simulink model "Computer"  (R2018b)
settings: Solver=ode4  StartTime=0.0  StopTime=SimEndTime  FixedStep=TimeStep  RelTol=1e-3
model workspace (MATLAB code in the model file):
  | CON = Simulink.Parameter;
  | CON.DataType = 'Bus: Bus_CON';
  | CON.Value = Simulink.Bus.createMATLABStruct('Bus_CON');
undefined symbols (not defined in the file): computer_dt
settings Model: ParameterArgumentNames=CON  OrderedModelArguments=off  Creator=Ethan  LastModifiedBy=Ethan
settings ModelReferenceCC: ModelReferenceNumInstancesAllowed=Single

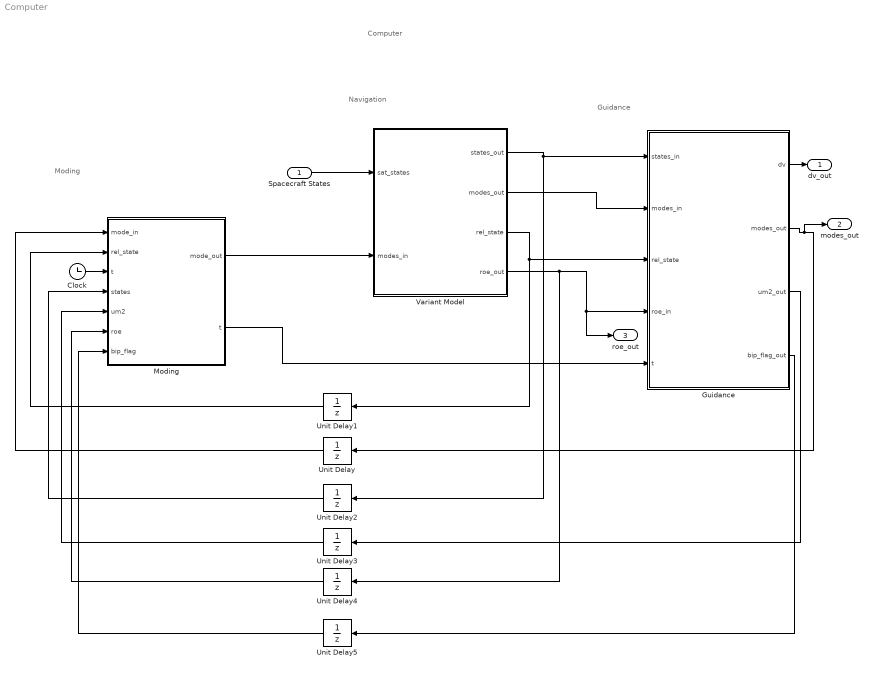
== system Computer ==
  note: Navigation
  note: Computer
  note: Moding
  note: Guidance
  Spacecraft States : Inport  OutDataTypeStr=Bus: Bus_outputs
  Clock : Clock
  Guidance : MATLAB Function  TreatAsAtomicUnit=on  SystemSampleTime=computer_dt
  Moding : MATLAB Function  TreatAsAtomicUnit=on  SystemSampleTime=computer_dt
  Unit Delay{,1..5} (6 alike) : UnitDelay  SampleTime=-1
  Variant Model : Subsystem  Variant=on
  dv_out : Outport  PortDimensions=3
  modes_out : Outport  Port=2  OutDataTypeStr=Bus: Bus_modes
  roe_out : Outport  Port=3  OutDataTypeStr=Bus: Bus_roe
  wires:
  Spacecraft States/1 -> Variant Model/1(sat_states)
  Variant Model/1(states_out) -> Unit Delay2/1, Guidance/1(states_in)
  Guidance/1(dv) -> dv_out/1
  Clock/1 -> Moding/3("t ")
  Moding/1(mode_out) -> Variant Model/2(modes_in)
  Variant Model/2(modes_out) -> Guidance/2(modes_in)
  Guidance/2(modes_out) -> modes_out/1, Unit Delay/1
  Unit Delay/1 -> Moding/1(mode_in)
  Variant Model/3(rel_state) -> Guidance/3(rel_state), Unit Delay1/1
  Unit Delay1/1 -> Moding/2(rel_state)
  Variant Model/4(roe_out) -> Unit Delay4/1, roe_out/1, Guidance/4(roe_in)
  Unit Delay2/1 -> Moding/4(states)
  Guidance/3(um2_out) -> Unit Delay3/1
  Unit Delay3/1 -> Moding/5(um2)
  Unit Delay4/1 -> Moding/6(roe)
  Moding/2(t) -> Guidance/5(t)
  Guidance/4(bip_flag_out) -> Unit Delay5/1
  Unit Delay5/1 -> Moding/7(bip_flag)

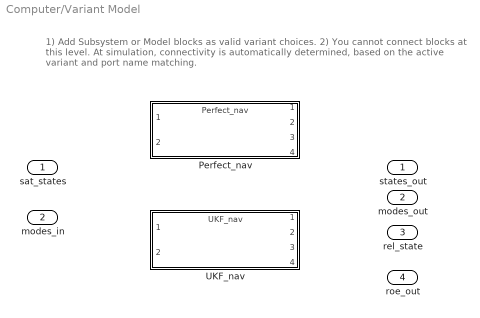
== system Computer/Variant Model ==
  note: 1) Add Subsystem or Model blocks as valid variant choices.
      | 2) You cannot connect blocks at this level. At simulation, connectivity is automatically
      | determined, based on the active variant and port name matching.
  sat_states : Inport  OutDataTypeStr=Bus: Bus_outputs
  modes_in : Inport  Port=2  OutDataTypeStr=Bus: Bus_modes
  Perfect_nav : ModelReference  DisableCoverage=on  ModelNameDialog=Perfect_nav  ParameterArgumentNames=CON  ParameterArgumentValues=CON  UsingDefaultArgumentValue=0  SimulationMode=Normal  VariantControl=Nav_variant  ModelReferenceVersion=1.97
  UKF_nav : ModelReference  ModelNameDialog=UKF_nav  ParameterArgumentNames=CON  ParameterArgumentValues=CON  UsingDefaultArgumentValue=0  SimulationMode=Normal  VariantControl=UKF_variant  ModelReferenceVersion=1.166
  states_out : Outport  OutDataTypeStr=Bus: Bus_outputs
  modes_out : Outport  Port=2  OutDataTypeStr=Bus: Bus_modes
  rel_state : Outport  Port=3
  roe_out : Outport  Port=4  OutDataTypeStr=Bus: Bus_roe

== matlab function Computer/Guidance ==
  data: states_in input; modes_in input Bus: Bus_modes; rel_state input; roe_in input; t input; dv output; CON parameter; modes_out output Bus: Bus_modes; um2_out output; bip_flag_out output
function [dv, modes_out, um2_out, bip_flag_out] = guid_bound_motion(states_in, modes_in, rel_state, roe_in, t, CON)
modes_out = modes_in;
dv = zeros(3, 1);
chief = states_in.NXS_out;
deputy = states_in.astro_out;
i2lvlh = rv2RTN(deputy.r_i, deputy.v_i);

persistent dv_old dv2 um2 xi bip_flag hold_start da de
if isempty(dv_old)
    dv_old = zeros(3, 1);
    dv2 = zeros(3, 1);
    um2 = 999;
    xi = 1000;
    bip_flag = 0;
    hold_start = 0;
    da = -10000;
    de = zeros(2,1);
end

%% New ROE Guidance
if modes_in.guid == 1 % go to 0.5 km relative
    
    [a_c] = ECI2OE(chief.r_i, chief.v_i, CON.mu);
    [~, ~, ~, ~, ~, ~, ud] = ECI2OE(deputy.r_i, deputy.v_i, CON.mu);
    %     if da == -10000
    da = -roe_in.da + 0.491/a_c;
    de = [-roe_in.dey;-roe_in.dex];
    %     end
    %     de = [0; 0];
    if xi == 1000
        xi = atan2(de(2), de(1));
        if xi < 0
            xi = xi + 2 * pi;
        end
    end
    
    um2 = xi + pi;
    if um2 > 2 * pi
        um2 = um2 - 2 * pi;
    elseif um2 < 0
        um2 = um2 + 2 * pi;
    end
    if dv_old ~= zeros(3, 1)
        modes_out.guid = 2;
        dv = zeros(3, 1);
    else
        if abs(ud * pi/180 - xi) < 1e-4
            [dv1_t, dv2_t] = opt_burn_roe(da, de, sqrt(CON.mu/a_c^3), a_c);
            dv = i2lvlh' * [0; dv1_t; 0];
            dv2 = [0; dv2_t; 0];
            da = -10000;
        end
    end
elseif modes_in.guid == 2
    if dv_old == zeros(3,1)
        modes_out.guid = 3;
    end
elseif modes_in.guid == 4
    if dv_old ~= zeros(3, 1)
        modes_out.guid = 5;
        dv = zeros(3, 1);
        xi = 1000;
    else
        dv = i2lvlh' * dv2;
        dv2 = zeros(3, 1);
    end
elseif modes_in.guid == 6
    [a_c] = ECI2OE(chief.r_i, chief.v_i, CON.mu);
    [~, ~, ~, ~, ~, ~, ud] = ECI2OE(deputy.r_i, deputy.v_i, CON.mu);

    de = [-roe_in.dey;-roe_in.dex];
    da = -roe_in.da;

    
    if xi == 1000
        xi = atan2(de(2), de(1));
        if xi < 0
            xi = xi + 2 * pi;
        end
    end
    um2 = xi + pi;
    
    if um2 > 2 * pi
        um2 = um2 - 2 * pi;
    elseif um2 < 0
        um2 = um2 + 2 * pi;
    end
    
    if dv_old ~= zeros(3, 1)
        modes_out.guid = 7;
        dv = zeros(3, 1);
    else
        if abs(ud * pi/180 - xi) < 1e-4
            [dv1_t, dv2_t] = opt_burn_roe(da, de, sqrt(CON.mu/a_c^3), a_c);
            dv = i2lvlh' * [0; dv1_t; 0];
            dv2 = [0; dv2_t; 0];
        end
    end
    
elseif modes_in.guid == 7
    if dv_old == zeros(3,1)
        modes_out.guid = 8;
    end
    
elseif modes_in.guid == 9
    if dv_old ~= zeros(3, 1)
        modes_out.guid = 10;
        dv = zeros(3, 1);
    else
        dv = i2lvlh' * dv2;
        dv2 = zeros(3, 1);
        xi = 1000;
    end
elseif modes_in.guid == 11 %Vbar approach
    [a_c, ~, ~, ~, ~, ~, uc] = ECI2OE(chief.r_i, chief.v_i, CON.mu);
    [~, ~, ~, ~, ~, ~, ud] = ECI2OE(deputy.r_i, deputy.v_i, CON.mu);
    if bip_flag == 0 && (t - hold_start) > 600

        da = -roe_in.da + 1e-10/a_c;
        dL = -roe_in.dL;
%         dL = -roe_in.dL;
        de = [0;0];
%         de = [-roe_in.dey;-roe_in.dex];
        if xi == 1000
            xi = atan2(de(2), de(1));
            if xi < 0
                xi = xi + 2 * pi;
            end
        end
        [dv_out, um2] = two_burn_roe(da, norm(de), dL, pi/180*ud, a_c, CON.mu, xi);
%         dv_out = [1e-13; 0; -1e-13; 0];
%         dv_out = [0; 1e-13; 0; -1e-13];
%         um2 = uc * pi/180 + pi*0.9;
        if um2 > 2*pi
            um2 = um2 - 2 * pi;
        end
        dv = i2lvlh' * [dv_out(1); dv_out(2); 0];
        dv2 = [dv_out(3); dv_out(4); 0];
        bip_flag = 1;
        
    elseif bip_flag && abs(ud * pi/180 - um2) < 1e-3
        dv = i2lvlh' * dv2;
        dv2 = zeros(3, 1);
        xi = 1000;
        hold_start = t;
        bip_flag = 0;
        modes_out.guid = 12;
    end
    
end


dv_old = dv;
um2_out = um2;
bip_flag_out = bip_flag;
end


%  [a_c, ~, ~, ~, ~, ~, uc] = ECI2OE(chief.r_i, chief.v_i, CON.mu);
%     if bip_flag == 0 && (t - hold_start) > 600
% %         if abs(rel_state(2)) < 0.07
% %             rel_state(2) = 0;
% %         end
%         %         if da == -10000
%         da = -roe_in.da + rel_state(2)/(1 * a_c);
%         %             da = -roe_in.da;
%         %             de = [-roe_in.dey-0.00001;-roe_in.dex-0.00001];
%         %         end
%         da = 0;
%         de = [-roe_in.dey;-roe_in.dex];
%         %     de = [0; 0];
%         if xi == 1000
%             xi = atan2(de(2), de(1));
%             if xi < 0
%                 xi = xi + 2 * pi;
%             end
%         end
%         
%         um2 = xi + pi;
%         if um2 > 2 * pi
%             um2 = um2 - 2 * pi;
%         elseif um2 < 0
%             um2 = um2 + 2 * pi;
%         end
%         
%         if abs(uc * pi/180 - xi) < 1e-4
%             [dv1_t, dv2_t] = opt_burn_roe(da, de, sqrt(CON.mu/a_c^3), a_c);
%             dv = i2lvlh' * [0; dv1_t; 0];
%             dv2 = [0; dv2_t; 0];
%             da = -10000;
%             bip_flag = 1;
%         end
%         
%     elseif bip_flag && abs(uc * pi/180 - um2) < 1e-3
%         dv = i2lvlh' * dv2;
%         dv2 = zeros(3, 1);
%         xi = 1000;
%         hold_start = t;
%         bip_flag = 0;
%     end

== matlab function Computer/Moding ==
  data: mode_in input Bus: Bus_modes; rel_state input; mode_out output Bus: Bus_modes; t input; states input; um2 input; roe input; CON parameter; t output; bip_flag input
function [mode_out, t] = moding(mode_in, rel_state, t, states, um2, roe, CON, bip_flag)

mode_out  = mode_in;
persistent tig_time
if isempty(tig_time)
    tig_time = 0;
end
chief = states.NXS_out;
deputy = states.astro_out;
a_c = ECI2OE(chief.r_i, chief.v_i, CON.mu);
[~, ~, ~, ~, ~, ~, ang] = ECI2OE(deputy.r_i, deputy.v_i, CON.mu);
da2 = 1000;
if CON.guidFlag == 1 && any(rel_state ~= zeros(6, 1))
    if rel_state(2) < 40 && mode_in.guid == 0 && t > 50
        mode_out.guid = 1;
    elseif (mode_in.guid == 3 || mode_in.guid == 8) && (abs(ang*pi/180 - um2) < 1e-3)
        mode_out.guid = mode_in.guid + 1;
    elseif mode_in.guid == 5 || mode_out.guid == 6
        if rel_state(2) < 9.3
            mode_out.guid = 6;
        end
    elseif mode_in.guid == 10
        if tig_time == 0
            tig_time = t;
        end
        if t - tig_time > 0
            mode_out.guid = 12;
        end
    elseif mode_in.guid == 11 && abs(rel_state(2)) < 0.05 && bip_flag == 0
        mode_out.guid = 12;
    end
end
